simulink model "e09"  (R2023b)
settings: Solver=FixedStepAuto  StartTime=0.0  StopTime=50  FixedStep=1e-4  RelTol=1e-3
values from neighbouring files (symbols this model uses):
  A1 = [ ... (first row only)    [e00.m]
  B1 = [0;0;g]    [e00.m]
  C1 = [0,1,0]    [e00.m]
  D1 = 0    [e00.m]
  kp = 0.17    [e00.m]
  td = 38    [e00.m]
  ti = 100    [e00.m]
settings Model: Creator=jitbitan  LastModifiedBy=Anirvan Krishna

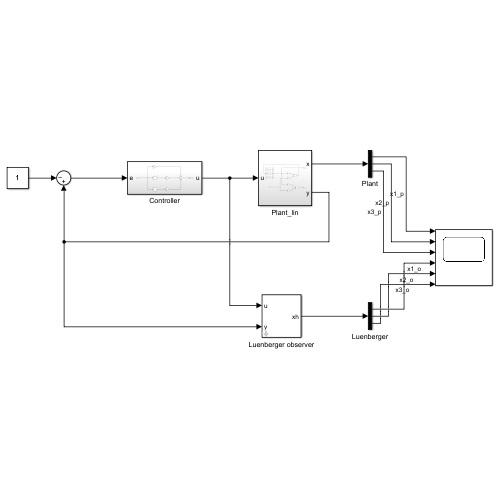
[thumbnail: Simulink's stored preview of the top-level diagram]
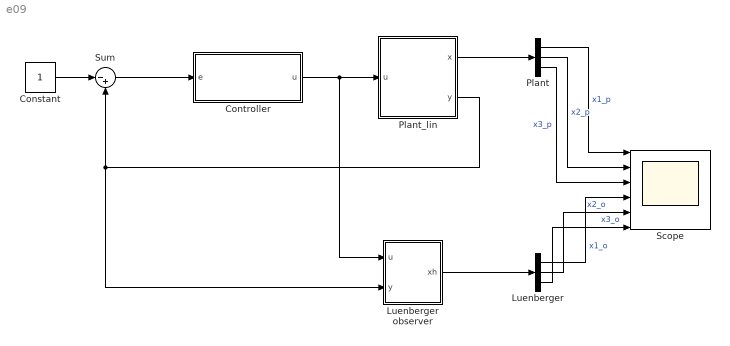
== system e09 ==
  Constant : Constant
  Controller : Subsystem
  Luenberger : Demux  Outputs=3
  Luenberger observer : Subsystem  mask{LuG=100}
      mask prompts: LuG "Luenberger Gain"
  Plant : Demux  Outputs=3
  Plant_lin : Subsystem
  Scope : Scope  NumInputPorts=6
  Sum : Sum  Inputs=|-+
  wires:
  Constant/1 -> Sum/1
  Controller/1(u) -> Plant_lin/1(u), Luenberger observer/1(u)
  Sum/1 -> Controller/1(e)
  Luenberger observer/1(xh) -> Luenberger/1
  Plant_lin/2(y) -> Sum/2, Luenberger observer/2(y)
  Plant_lin/1(x) -> Plant/1
  Plant/1 -> Scope/1  "x1_p"
  Luenberger/1 -> Scope/4  "x1_o"
  Plant/2 -> Scope/2  "x2_p"
  Plant/3 -> Scope/3  "x3_p"
  Luenberger/2 -> Scope/5  "x2_o"
  Luenberger/3 -> Scope/6  "x3_o"

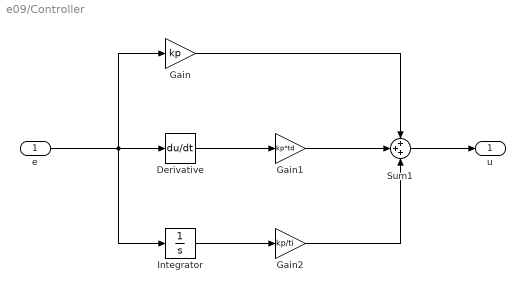
== system e09/Controller ==
  e : Inport
  Derivative : Derivative
  Gain : Gain  Gain=kp
  Gain1 : Gain  Gain=kp*td
  Gain2 : Gain  Gain=kp/ti
  Integrator : Integrator
  Sum1 : Sum  Inputs=+++
  u : Outport
  wires:
  e/1 -> Derivative/1, Integrator/1, Gain/1
  Sum1/1 -> u/1
  Gain/1 -> Sum1/1
  Derivative/1 -> Gain1/1
  Gain1/1 -> Sum1/2
  Integrator/1 -> Gain2/1
  Gain2/1 -> Sum1/3

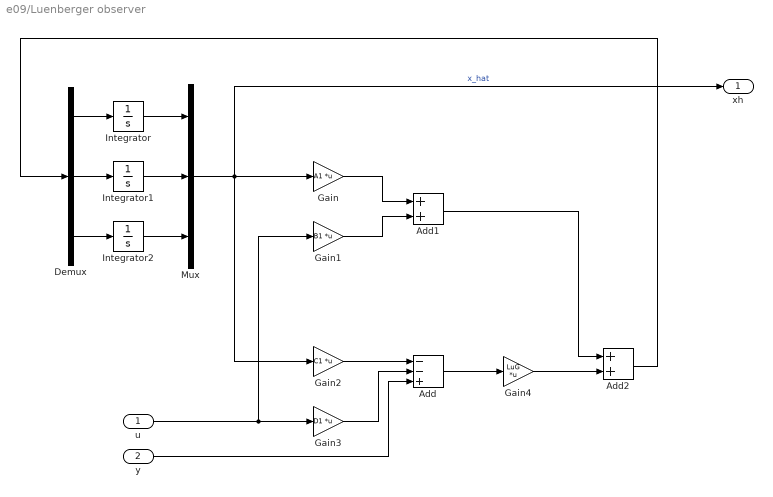
== system e09/Luenberger observer ==
  u : Inport
  y : Inport  Port=2
  Add : Sum  Inputs=--+
  Add1 : Sum
  Add2 : Sum
  Demux : Demux  Outputs=3
  Gain : Gain  Gain=A1  Multiplication=Matrix(K*u)
  Gain1 : Gain  Gain=B1  Multiplication=Matrix(K*u)
  Gain2 : Gain  Gain=C1  Multiplication=Matrix(K*u)
  Gain3 : Gain  Gain=D1  Multiplication=Matrix(K*u)
  Gain4 : Gain  Gain=LuG  Multiplication=Matrix(K*u)
  Integrator : Integrator
  Integrator1 : Integrator
  Integrator2 : Integrator
  Mux : Mux  Inputs=3
  xh : Outport
  wires:
  Integrator2/1 -> Mux/3
  Mux/1 -> Gain2/1, Gain/1, xh/1  "x_hat"
  Demux/1 -> Integrator/1
  Gain1/1 -> Add1/2
  Demux/2 -> Integrator1/1
  Demux/3 -> Integrator2/1
  Add/1 -> Gain4/1
  u/1 -> Gain1/1, Gain3/1
  Gain/1 -> Add1/1
  Add2/1 -> Demux/1
  Gain3/1 -> Add/2
  Gain2/1 -> Add/1
  Add1/1 -> Add2/1
  Gain4/1 -> Add2/2
  Integrator/1 -> Mux/1
  Integrator1/1 -> Mux/2
  y/1 -> Add/3

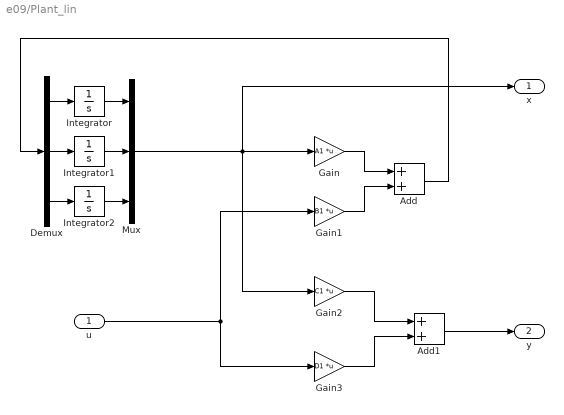
== system e09/Plant_lin ==
  u : Inport
  Add : Sum
  Add1 : Sum
  Demux : Demux  Outputs=3
  Gain : Gain  Gain=A1  Multiplication=Matrix(K*u)
  Gain1 : Gain  Gain=B1  Multiplication=Matrix(K*u)
  Gain2 : Gain  Gain=C1  Multiplication=Matrix(K*u)
  Gain3 : Gain  Gain=D1  Multiplication=Matrix(K*u)
  Integrator : Integrator
  Integrator1 : Integrator
  Integrator2 : Integrator
  Mux : Mux  Inputs=3
  x : Outport
  y : Outport  Port=2
  wires:
  Gain2/1 -> Add1/1
  Gain3/1 -> Add1/2
  Demux/1 -> Integrator/1
  Integrator2/1 -> Mux/3
  Demux/3 -> Integrator2/1
  Integrator1/1 -> Mux/2
  Demux/2 -> Integrator1/1
  Gain/1 -> Add/1
  Add/1 -> Demux/1
  Integrator/1 -> Mux/1
  Gain1/1 -> Add/2
  u/1 -> Gain3/1, Gain1/1
  Mux/1 -> Gain2/1, Gain/1, x/1
  Add1/1 -> y/1
